simulink model "MPC_plant"  (R2024b)
settings: Solver=ode45  StartTime=0.0  StopTime=400  RelTol=1e-2  EnableMultiTasking=on
values from neighbouring files (symbols this model uses):
  alfa = [alfaa alfab alfac alfad alfae alfaf]    [dati.m]
  F0B = 0.5    [dati.m]
  F0E = u(10)    [R2_stati.m]    (also in dati.m = 99.5)
  H1 = [Hr1;He1*ones(Ne1,1);Hf1;Ha1*ones(Na1,1);Hc1]    [dati.m]
  H2 = [Hr2;He2*ones(Ne2,1);Hf2;Ha2*ones(Na2,1);Hc2]    [dati.m]
  H3 = [Hr3;He3*ones(Ne3,1);Hf3;Ha3*ones(Na3,1);Hc3]    [dati.m]
  k1 = 10    [dati.m]
  k2 = 50    [dati.m]
  N1 = Na1+Ne1+3    (= 9)    [dati.m]
  N2 = Na2+Ne2+3    (= 9)    [dati.m]
  N3 = Na3+Ne3+3    (= 9)    [dati.m]
  Na1 = 3    [dati.m]
  Na2 = 3    [dati.m]
  Na3 = 3    [dati.m]
  Ne1 = 3    [dati.m]
  Ne2 = 3    [dati.m]
  Ne3 = 3    [dati.m]
  V1 = 330+80    (= 410)    [dati.m]
  V2 = 385    [dati.m]
  V3 = 282    [dati.m]
  VR1 = 1000    [dati.m]
  VR2 = 850    [dati.m]
  x1a = zeros(N1,1)    [dati.m]
  x1b = zeros(N1,1)    [dati.m]
  x1c = zeros(N1,1)    [dati.m]
  x2a = zeros(N2,1)    [dati.m]
  x2b = zeros(N2,1)    [dati.m]
  x2c = zeros(N2,1)    [dati.m]
  x3a = zeros(N3,1)    [dati.m]
  x3b = zeros(N3,1)    [dati.m]
  x3c = zeros(N3,1)    [dati.m]
  xD3_a = 0.    (= 0)    [dati.m]
  xD3_c = 0.0036    [dati.m]
  xD3_d = 0.2817    [dati.m]
  xk0_obs = 0.5*ones(states_tot, 1)    [Initialize_forequilibrium.m]    (also in MPC_main.m)
  z0A_a = 1    [dati.m]
  z0A_b = 0    [dati.m]
  z0A_c = 0    [dati.m]
  z0A_d = 0    [dati.m]
  z0B_a = 0    [dati.m]
  z0B_b = 1    [dati.m]
  z0B_c = 0    [dati.m]
  z0B_d = 0    [dati.m]
  z0E_b = 0    [dati.m]
  z0E_d = 0    [dati.m]
  z0E_e = 1    [dati.m]
  z0E_f = 0    [dati.m]
  z1a = 0.184    [dati.m]
  z1b = 0.0544    [dati.m]
  z1c = 0.3255    [dati.m]
  z1d = 0.4361    [dati.m]
  z2b = u(4)    [R2_stati.m]    (also in R3_stati.m = u(9); dati.m = 0.4455)
  z2d = u(1)    [R2_stati.m]    (also in R3_stati.m = u(6); dati.m = 0.0514)
  z2e = u(2)    [R2_stati.m]    (also in R3_stati.m = u(7); dati.m = 0.0411)
  z2f = u(3)    [R2_stati.m]    (also in R3_stati.m = u(8); dati.m = 0.4455)
  z3b = u(4)    [R3_stati.m]    (also in dati.m = 0.4666)
  z3d = u(1)    [R3_stati.m]    (also in dati.m = 0.0523)
  z3e = u(2)    [R3_stati.m]    (also in dati.m = 0.0032)
  z3f = u(3)    [R3_stati.m]    (also in dati.m = 0.4666)
undefined symbols (not defined in the file or in its folder): colonna1, colonna2, colonna3, R1_portata, R1_stati, R2_portata, R2_stati, R3_portata, R3_stati, somma
settings Model: Creator=scattolini  LastModifiedBy=Laura
settings SolverCC: AlgebraicLoopSolver=TrustRegion
settings DataIOCC: LimitDataPoints=on  SaveFormat=Array  SignalLoggingSaveFormat=ModelDataLogs  ReturnWorkspaceOutputs=off
settings OptimizationCC: BlockReduction=off  DefaultParameterBehavior=Inlined  InlineInvariantSignals=on  BufferReuse=off  ExpressionDepthLimit=2147483647  InitFltsAndDblsToZero=on  LifeSpan=inf
settings DebuggingCC: SaveWithParameterizedLinksMsg=none  UnderspecifiedInitializationDetection=Classic  MergeDetectMultiDrivingBlocksExec=none  SignalResolutionControl=TryResolveAllWithWarning  SolverPrmCheckMsg=warning  MultiTaskDSMMsg=warning  MultiTaskCondExecSysMsg=none  FcnCallInpInsideContextMsg=warning  UnconnectedInputMsg=warning  UnconnectedOutputMsg=warning  UnconnectedLineMsg=warning  StateNameClashWarn=warning  SFUnexpectedBacktrackingDiag=warning  SFNoUnconditionalDefaultTransitionDiag=warning  SFExecutionAtInitializationDiag=none  ArithmeticOperatorsInVariantConditions=warning
settings HardwareCC: ProdBitPerPointer=32  ProdBitPerSizeT=32  ProdBitPerPtrDiffT=32  ProdLargestAtomicFloat=None  ProdIntDivRoundTo=Undefined  ProdEndianess=Unspecified  ProdWordSize=32  ProdHWDeviceType=32-bit Generic
settings ModelReferenceCC: EnableRefExpFcnMdlSchedulingChecks=on  PropagateSignalLabelsOutOfModel=off
settings RTWCC: GPUComputeCapability=3.5  DLArmComputeVersion=19.05
settings CodeAppCC: StateflowObjectComments=on
settings GRTTargetCC: TargetFcnLib=ansi_tfl_tmw.mat  TargetLangStandard=C89/C90 (ANSI)  CombineOutputUpdateFcns=off  GRTInterface=on
settings ConfigComp: CovMetricSettings=dw  CovSaveCumulativeToWorkspaceVar=on  CovSaveSingleToWorkspaceVar=on

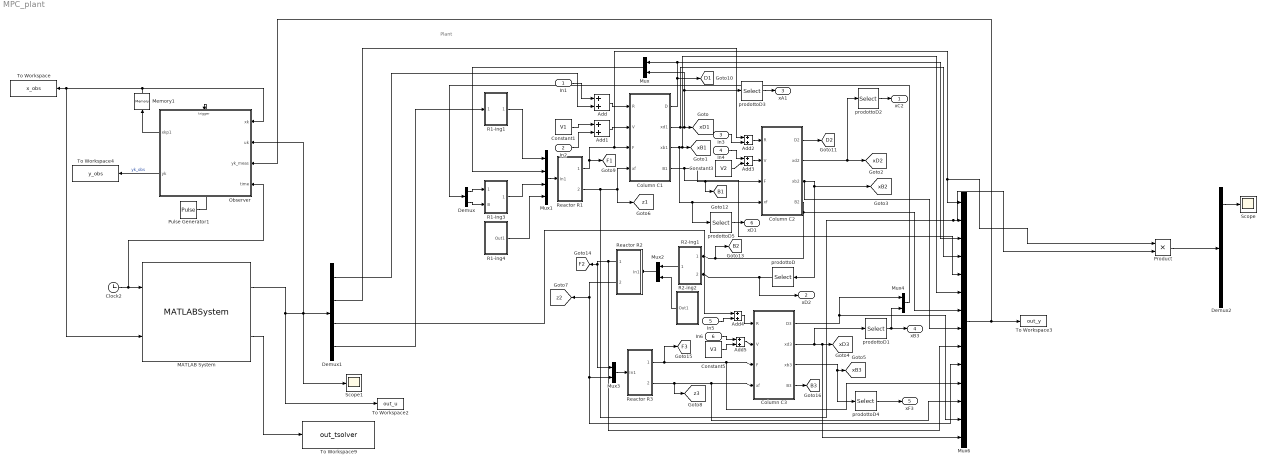
== system MPC_plant ==
  note: Plant
  In1 : Inport
  In2 : Inport  Port=2
  In3 : Inport  Port=3
  In4 : Inport  Port=4
  In5 : Inport  Port=5
  In6 : Inport  Port=6
  Add{,1..5} (6 alike) : Sum
  Clock2 : Clock
  Column C1 : Subsystem
  Column C2 : Subsystem
  Column C3 : Subsystem
  Constant1 : Constant  Value=V1
  Constant3 : Constant  Value=V2
  Constant5 : Constant  Value=V3
  Demux : Demux  Outputs=2
  Demux1 : Demux
  Demux2 : Demux
  MATLAB System : MATLABSystem  System=MPC_function  tau_s=1  N=12  T_s=1  T_b=1  SimulateUsing=Interpreted execution
      mask Type: MPC_function
      mask Display:
      | disp('MPC_function');
      | port_label('input',1,'t');
      | port_label('input',2,'xk');
      | port_label('output',1,'u_opt');
      | port_label('output',2,'t_solver');
  Memory1 : Memory  InitialCondition=xk0_obs
  Mux{,2..4} (4 alike) : Mux  Inputs=2
  Mux1 : Mux
  Mux6 : Mux  Inputs=14
  Observer : Subsystem  TreatAsAtomicUnit=on
  Product : Product
  Pulse Generator1 : DiscretePulseGenerator  PulseType=Time based  Period=1  PulseWidth=5
  R1-ing1 : Subsystem
  R1-ing3 : Subsystem
  R1-ing4 : Subsystem
  R2-ing1 : Subsystem
  R2-ing2 : Subsystem
  Reactor R1 : Subsystem
  Reactor R2 : Subsystem
  Reactor R3 : Subsystem
  Scope : Scope
  Scope1 : Scope
  To Workspace : ToWorkspace  VariableName=x_obs  SampleTime=1
  To Workspace2 : ToWorkspace  VariableName=out_u  SampleTime=1
  To Workspace3 : ToWorkspace  VariableName=out_y  SampleTime=1
  To Workspace4 : ToWorkspace  VariableName=y_obs  SampleTime=1
  To Workspace9 : ToWorkspace  VariableName=out_tsolver  SampleTime=1
  prodottoD : Selector  InputPortWidth=4  IndexOptions=Index vector (dialog)  Indices=4  OutputSizes=1
  prodottoD1 : Selector  InputPortWidth=4  IndexOptions=Index vector (dialog)  Indices=1  OutputSizes=1
  prodottoD2 : Selector  InputPortWidth=4  IndexOptions=Index vector (dialog)  Indices=3  OutputSizes=1
  prodottoD3 : Selector  InputPortWidth=4  IndexOptions=Index vector (dialog)  Indices=1  OutputSizes=1
  prodottoD4 : Selector  InputPortWidth=4  IndexOptions=Index vector (dialog)  Indices=4  OutputSizes=1
  prodottoD5 : Selector  InputPortWidth=4  IndexOptions=Index vector (dialog)  Indices=4  OutputSizes=1
  xC2 : Outport
  xD2 : Outport  Port=2
  xA1 : Outport  Port=3
  xB3 : Outport  Port=4
  xF3 : Outport  Port=5
  xD1 : Outport  Port=6
  tag scope: B1=global, B2=global, B3=global, D1=global, D2=global, F1=global, F2=global, F3=global, xB1=global, xB2=global, xB3=global, xD1=global, xD2=global, xD3=global, z1=global, z2=global, z3=global
  wires:
  R1-ing1/1(Out1) -> Mux1/1
  R1-ing3/1(Out1) -> Mux1/3
  R1-ing4/1(Out1) -> Mux1/4
  Mux1/1 -> Reactor R1/1(In1)
  Column C1/3(xb1) -> Mux6/6, [xB1], Column C2/4(xf), prodottoD5/1
  Column C1/2(xd1) -> Mux6/4, [xD1], Mux/2, prodottoD3/1
  Column C1/1(D) -> Mux6/3, Mux/1, [D1]
  Mux/1 -> Mux1/2
  Column C1/4(B1) -> Mux6/5, Column C2/3(F), [B1]
  prodottoD/1 -> R2-ing1/2(prodottoD), xD2/1
  Mux2/1 -> Reactor R2/1(In1)
  R2-ing1/1(Out1) -> Mux2/1
  R2-ing2/1(Out1) -> Mux2/2
  Reactor R2/2(stati) -> Mux6/10, Mux3/2, [z2]
  Reactor R2/1(portata) -> Mux6/9, Mux3/1, [F2]
  Mux3/1 -> Reactor R3/1(In1)
  Reactor R3/1(portata) -> Mux6/11, Column C3/3(F), [F3]
  Reactor R3/2(stati B-D-E-F) -> Mux6/12, Column C3/4(xf), [z3]
  Column C3/3(xb3) -> [xB3], prodottoD4/1
  Column C3/2(xd3) -> Mux6/14, [xD3], prodottoD1/1
  Column C2/2(xd2) -> [xD2], prodottoD2/1
  Column C2/1(D2) -> [D2]
  prodottoD1/1 -> Mux4/2, xB3/1
  Column C3/1(D3) -> Mux4/1, Mux6/13
  Mux4/1 -> Demux/1
  Demux/1 -> R1-ing3/1(portata)
  Demux/2 -> R1-ing3/2(B)
  Demux1/1 -> Add/2
  In1/1 -> Add/1
  Add/1 -> Column C1/1(R)
  prodottoD2/1 -> xC2/1
  Add1/1 -> Column C1/2(V)
  Constant1/1 -> Add1/1
  In2/1 -> Add1/2
  Add2/1 -> Column C2/1(R)
  Add3/1 -> Column C2/2(V)
  Constant3/1 -> Add3/2
  In3/1 -> Add2/2
  In4/1 -> Add3/1
  prodottoD3/1 -> xA1/1
  Add5/1 -> Column C3/2(V)
  Constant5/1 -> Add5/2
  In6/1 -> Add5/1
  In5/1 -> Add4/2
  prodottoD4/1 -> xF3/1
  Column C3/4(B3) -> [B3]
  Add4/1 -> Column C3/1(R)
  prodottoD5/1 -> xD1/1
  Mux6/1 -> Observer/3(yk_meas), To Workspace3/1
  Pulse Generator1/1 -> Observer/Trigger
  Observer/1(xkp1) -> Memory1/1
  Memory1/1 -> Observer/1(xk), To Workspace/1, MATLAB System/2
  Observer/2(yk) -> To Workspace4/1  "yk_obs"
  Column C2/3(xb2) -> Mux6/8, prodottoD/1, [xB2]
  Column C2/4(B2) -> Mux6/7, R2-ing1/1(portataD), [B2]
  Clock2/1 -> Observer/4(time), MATLAB System/1
  Demux1/2 -> Add2/1
  Demux1/3 -> Add4/1
  Demux1/4 -> R1-ing1/1(F0A)
  Reactor R1/1(portata) -> Mux6/1, Product/1, Column C1/3(F), [F1]
  Reactor R1/2(stati) -> Product/2, Mux6/2, Column C1/4(xf), [z1]
  Product/1 -> Demux2/1
  Demux2/1 -> Scope/1
  MATLAB System/1 -> To Workspace2/1, Demux1/1, Observer/2(uk), Scope1/1
  MATLAB System/2 -> To Workspace9/1

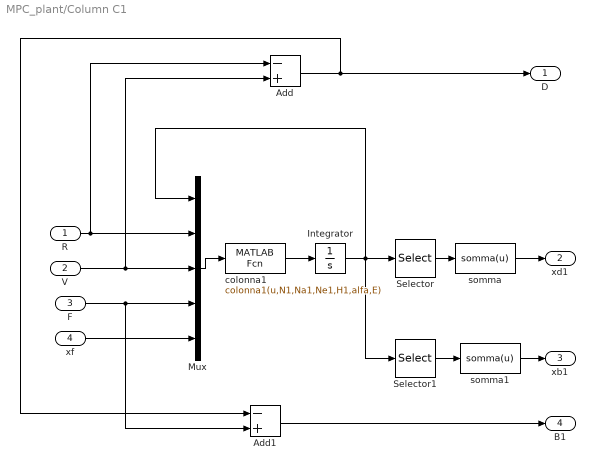
== system MPC_plant/Column C1 ==
  R : Inport
  V : Inport  Port=2
  F : Inport  Port=3
  xf : Inport  Port=4
  Add : Sum  Inputs=-+
  Add1 : Sum  Inputs=-+
  Integrator : Integrator  InitialCondition=[x1a;x1b;x1c]
  Mux : Mux  Inputs=5
  Selector : Selector  InputPortWidth=N1*3  IndexOptions=Index vector (dialog)  Indices=[N1 2*N1 3*N1]  OutputSizes=1
  Selector1 : Selector  InputPortWidth=N1*3  IndexOptions=Index vector (dialog)  Indices=[1 N1+1 2*N1+1]  OutputSizes=1
  colonna1 : MATLABFcn  MATLABFcn=colonna1(u,N1,Na1,Ne1,H1,alfa,E)  OutputDimensions=N1*3
  somma : MATLABFcn  MATLABFcn=somma(u)  OutputDimensions=4
  somma1 : MATLABFcn  MATLABFcn=somma(u)  OutputDimensions=4
  D : Outport
  xd1 : Outport  Port=2
  xb1 : Outport  Port=3
  B1 : Outport  Port=4
  wires:
  Mux/1 -> colonna1/1
  colonna1/1 -> Integrator/1
  Integrator/1 -> Selector/1, Mux/1, Selector1/1
  R/1 -> Mux/2, Add/1
  V/1 -> Mux/3, Add/2
  F/1 -> Mux/4, Add1/2
  xf/1 -> Mux/5
  Selector/1 -> somma/1
  somma/1 -> xd1/1
  Selector1/1 -> somma1/1
  somma1/1 -> xb1/1
  Add/1 -> D/1, Add1/1
  Add1/1 -> B1/1

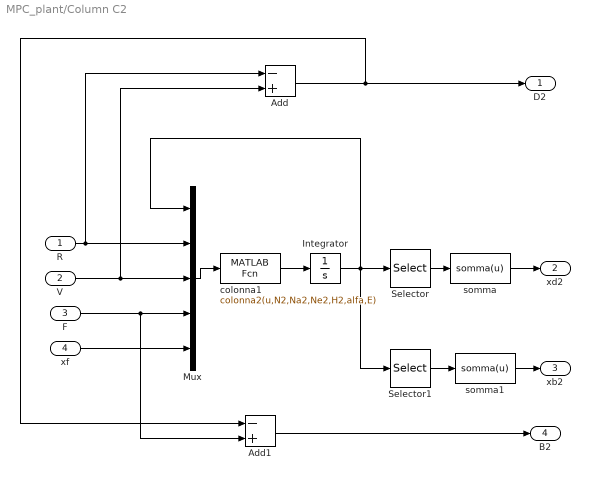
== system MPC_plant/Column C2 ==
  R : Inport
  V : Inport  Port=2
  F : Inport  Port=3
  xf : Inport  Port=4
  Add : Sum  Inputs=-+
  Add1 : Sum  Inputs=-+
  Integrator : Integrator  InitialCondition=[x2a;x2b;x2c]
  Mux : Mux  Inputs=5
  Selector : Selector  InputPortWidth=N2*3  IndexOptions=Index vector (dialog)  Indices=[N2 2*N2 3*N2]  OutputSizes=1
  Selector1 : Selector  InputPortWidth=N2*3  IndexOptions=Index vector (dialog)  Indices=[1 N2+1 2*N2+1]  OutputSizes=1
  colonna1 : MATLABFcn  MATLABFcn=colonna2(u,N2,Na2,Ne2,H2,alfa,E)  OutputDimensions=N2*3
  somma : MATLABFcn  MATLABFcn=somma(u)  OutputDimensions=4
  somma1 : MATLABFcn  MATLABFcn=somma(u)  OutputDimensions=4
  D2 : Outport
  xd2 : Outport  Port=2
  xb2 : Outport  Port=3
  B2 : Outport  Port=4
  wires:
  Mux/1 -> colonna1/1
  colonna1/1 -> Integrator/1
  Integrator/1 -> Selector/1, Mux/1, Selector1/1
  R/1 -> Mux/2, Add/1
  V/1 -> Mux/3, Add/2
  F/1 -> Mux/4, Add1/2
  xf/1 -> Mux/5
  Selector/1 -> somma/1
  somma/1 -> xd2/1
  Selector1/1 -> somma1/1
  somma1/1 -> xb2/1
  Add/1 -> D2/1, Add1/1
  Add1/1 -> B2/1

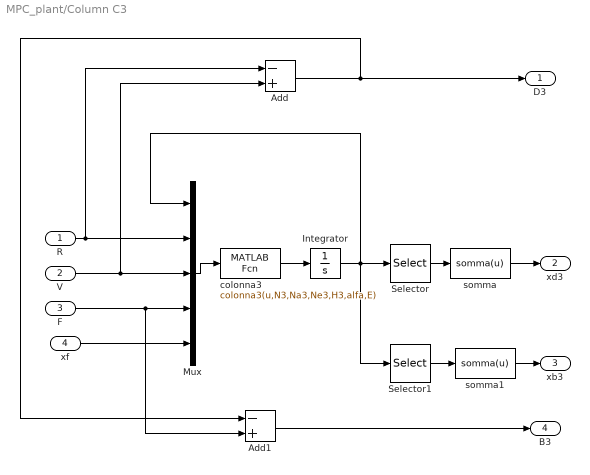
== system MPC_plant/Column C3 ==
  R : Inport
  V : Inport  Port=2
  F : Inport  Port=3
  xf : Inport  Port=4
  Add : Sum  Inputs=-+
  Add1 : Sum  Inputs=-+
  Integrator : Integrator  InitialCondition=[x3a;x3b;x3c]
  Mux : Mux  Inputs=5
  Selector : Selector  InputPortWidth=N3*3  IndexOptions=Index vector (dialog)  Indices=[N3 2*N3 3*N3]  OutputSizes=1
  Selector1 : Selector  InputPortWidth=N3*3  IndexOptions=Index vector (dialog)  Indices=[1 N3+1 2*N3+1]  OutputSizes=1
  colonna3 : MATLABFcn  MATLABFcn=colonna3(u,N3,Na3,Ne3,H3,alfa,E)  OutputDimensions=N3*3
  somma : MATLABFcn  MATLABFcn=somma(u)  OutputDimensions=4
  somma1 : MATLABFcn  MATLABFcn=somma(u)  OutputDimensions=4
  D3 : Outport
  xd3 : Outport  Port=2
  xb3 : Outport  Port=3
  B3 : Outport  Port=4
  wires:
  Mux/1 -> colonna3/1
  colonna3/1 -> Integrator/1
  Integrator/1 -> Selector/1, Mux/1, Selector1/1
  R/1 -> Mux/2, Add/1
  V/1 -> Mux/3, Add/2
  F/1 -> Mux/4, Add1/2
  xf/1 -> Mux/5
  Selector/1 -> somma/1
  somma/1 -> xd3/1
  Selector1/1 -> somma1/1
  somma1/1 -> xb3/1
  Add/1 -> D3/1, Add1/1
  Add1/1 -> B3/1

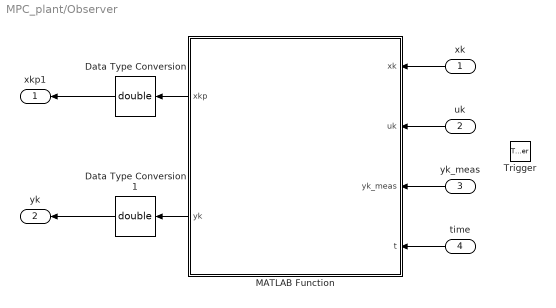
== system MPC_plant/Observer ==
  xk : Inport
  uk : Inport  Port=2
  yk_meas : Inport  Port=3
  time : Inport  Port=4
  Trigger : TriggerPort  VariantControl=(inherit)
  Data Type Conversion : DataTypeConversion  OutDataTypeStr=double  RndMeth=Nearest  SaturateOnIntegerOverflow=off
  Data Type Conversion1 : DataTypeConversion  OutDataTypeStr=double  RndMeth=Nearest  SaturateOnIntegerOverflow=off
  MATLAB Function : MATLAB Function  TreatAsAtomicUnit=on
  xkp1 : Outport
  yk : Outport  Port=2
  wires:
  xk/1 -> MATLAB Function/1(xk)
  uk/1 -> MATLAB Function/2(uk)
  MATLAB Function/2(yk) -> Data Type Conversion1/1
  MATLAB Function/1(xkp) -> Data Type Conversion/1
  Data Type Conversion/1 -> xkp1/1
  Data Type Conversion1/1 -> yk/1
  yk_meas/1 -> MATLAB Function/3(yk_meas)
  time/1 -> MATLAB Function/4(t)

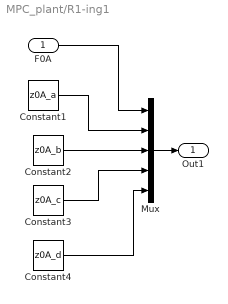
== system MPC_plant/R1-ing1 ==
  F0A : Inport
  Constant1 : Constant  Value=z0A_a
  Constant2 : Constant  Value=z0A_b
  Constant3 : Constant  Value=z0A_c
  Constant4 : Constant  Value=z0A_d
  Mux : Mux  Inputs=5
  Out1 : Outport
  wires:
  Constant1/1 -> Mux/2
  Constant2/1 -> Mux/3
  Constant3/1 -> Mux/4
  Constant4/1 -> Mux/5
  Mux/1 -> Out1/1
  F0A/1 -> Mux/1

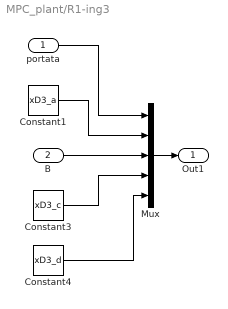
== system MPC_plant/R1-ing3 ==
  portata : Inport
  B : Inport  Port=2
  Constant1 : Constant  Value=xD3_a
  Constant3 : Constant  Value=xD3_c
  Constant4 : Constant  Value=xD3_d
  Mux : Mux  Inputs=5
  Out1 : Outport
  wires:
  portata/1 -> Mux/1
  Constant1/1 -> Mux/2
  B/1 -> Mux/3
  Constant3/1 -> Mux/4
  Constant4/1 -> Mux/5
  Mux/1 -> Out1/1

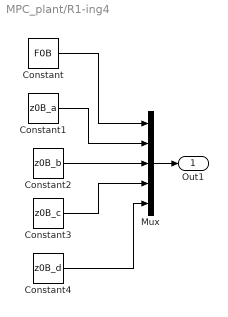
== system MPC_plant/R1-ing4 ==
  Constant : Constant  Value=F0B
  Constant1 : Constant  Value=z0B_a
  Constant2 : Constant  Value=z0B_b
  Constant3 : Constant  Value=z0B_c
  Constant4 : Constant  Value=z0B_d
  Mux : Mux  Inputs=5
  Out1 : Outport
  wires:
  Constant/1 -> Mux/1
  Constant1/1 -> Mux/2
  Constant2/1 -> Mux/3
  Constant3/1 -> Mux/4
  Constant4/1 -> Mux/5
  Mux/1 -> Out1/1

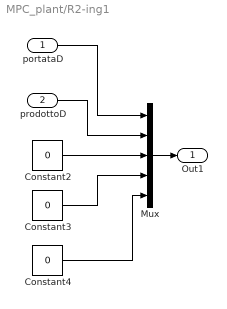
== system MPC_plant/R2-ing1 ==
  portataD : Inport
  prodottoD : Inport  Port=2
  Constant2 : Constant  Value=0
  Constant3 : Constant  Value=0
  Constant4 : Constant  Value=0
  Mux : Mux  Inputs=5
  Out1 : Outport
  wires:
  portataD/1 -> Mux/1
  prodottoD/1 -> Mux/2
  Constant2/1 -> Mux/3
  Constant3/1 -> Mux/4
  Constant4/1 -> Mux/5
  Mux/1 -> Out1/1

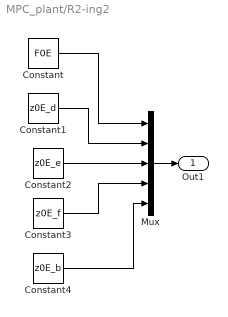
== system MPC_plant/R2-ing2 ==
  Constant : Constant  Value=F0E
  Constant1 : Constant  Value=z0E_d
  Constant2 : Constant  Value=z0E_e
  Constant3 : Constant  Value=z0E_f
  Constant4 : Constant  Value=z0E_b
  Mux : Mux  Inputs=5
  Out1 : Outport
  wires:
  Constant/1 -> Mux/1
  Constant1/1 -> Mux/2
  Constant2/1 -> Mux/3
  Constant3/1 -> Mux/4
  Constant4/1 -> Mux/5
  Mux/1 -> Out1/1

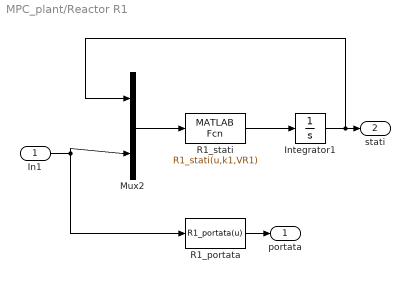
== system MPC_plant/Reactor R1 ==
  In1 : Inport
  Integrator1 : Integrator  InitialCondition=[z1a z1b z1c z1d]
  Mux2 : Mux  Inputs=2
  R1_portata : MATLABFcn  MATLABFcn=R1_portata(u)
  R1_stati : MATLABFcn  MATLABFcn=R1_stati(u,k1,VR1)  OutputDimensions=4
  portata : Outport
  stati : Outport  Port=2
  wires:
  In1/1 -> Mux2/2, R1_portata/1
  R1_stati/1 -> Integrator1/1
  Mux2/1 -> R1_stati/1
  Integrator1/1 -> Mux2/1, stati/1
  R1_portata/1 -> portata/1

== system MPC_plant/Reactor R2 ==
  In1 : Inport
  Integrator1 : Integrator  InitialCondition=[z2d z2e z2f z2b]
  Mux2 : Mux  Inputs=2
  R2_portata : MATLABFcn  MATLABFcn=R2_portata(u)
  R2_stati : MATLABFcn  MATLABFcn=R2_stati(u,k2,VR2)  OutputDimensions=4
  portata : Outport
  stati : Outport  Port=2
  wires:
  In1/1 -> Mux2/2, R2_portata/1
  R2_stati/1 -> Integrator1/1
  Mux2/1 -> R2_stati/1
  Integrator1/1 -> Mux2/1, stati/1
  R2_portata/1 -> portata/1

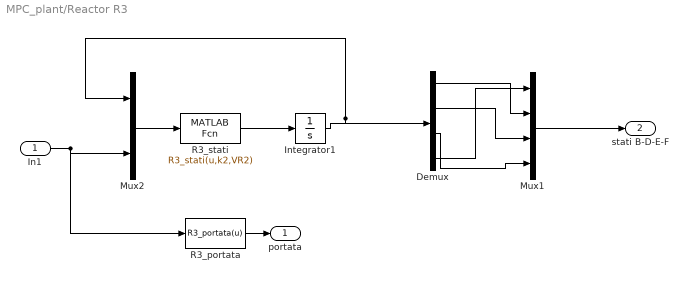
== system MPC_plant/Reactor R3 ==
  In1 : Inport
  Demux : Demux
  Integrator1 : Integrator  InitialCondition=[z3d z3e z3f z3b]
  Mux1 : Mux
  Mux2 : Mux  Inputs=2
  R3_portata : MATLABFcn  MATLABFcn=R3_portata(u)
  R3_stati : MATLABFcn  MATLABFcn=R3_stati(u,k2,VR2)  OutputDimensions=4
  portata : Outport
  stati B-D-E-F : Outport  Port=2
  wires:
  In1/1 -> Mux2/2, R3_portata/1
  R3_stati/1 -> Integrator1/1
  Mux2/1 -> R3_stati/1
  Integrator1/1 -> Mux2/1, Demux/1
  R3_portata/1 -> portata/1
  Demux/4 -> Mux1/1
  Demux/1 -> Mux1/2
  Demux/2 -> Mux1/3
  Demux/3 -> Mux1/4
  Mux1/1 -> stati B-D-E-F/1

== matlab function MPC_plant/Observer/MATLAB Function ==
  data: xkp output; xk input; uk input; yk_meas input; t input; yk output
function [xkp, yk] = RNN(xk, uk, yk_meas, t)

    if t <= 1
        xk = 0.5*ones(18, 1);
    end

    n_states = [3,3,3,3,3,3];
    layers_file = load("layers_file.mat");
    layers_file = layers_file.layers_file;
    input_scaler_bias = load("input_scaler_bias.mat");
    input_scaler_scale_common = load("input_scaler_scale_common.mat");
    output_scaler_bias = load("output_scaler_bias.mat");
    output_scaler_scale_common = load("output_scaler_scale_common.mat");
    
    % Best observer weight
    Lz1_sol = load("Lz1_sol.mat");
    Lf1_sol = load("Lf1_sol.mat");
    Lz1 = Lz1_sol.Lz1;
    Lf1 = Lf1_sol.Lf1;
    Lz2_sol = load("Lz2_sol.mat");
    Lf2_sol = load("Lf2_sol.mat");
    Lz2 = Lz2_sol.Lz2;
    Lf2 = Lf2_sol.Lf2;
    Lz3_sol = load("Lz3_sol.mat");
    Lf3_sol = load("Lf3_sol.mat");
    Lz3 = Lz3_sol.Lz3;
    Lf3 = Lf3_sol.Lf3;
    Lz4_sol = load("Lz4_sol.mat");
    Lf4_sol = load("Lf4_sol.mat");
    Lz4 = Lz4_sol.Lz4;
    Lf4 = Lf4_sol.Lf4;
    Lz5_sol = load("Lz5_sol.mat");
    Lf5_sol = load("Lf5_sol.mat");
    Lz5 = Lz5_sol.Lz5;
    Lf5 = Lf5_sol.Lf5;
    Lz6_sol = load("Lz6_sol.mat");
    Lf6_sol = load("Lf6_sol.mat");
    Lz6 = Lz6_sol.Lz6;
    Lf6 = Lf6_sol.Lf6;

    % Scale input and output
    uk = (uk  - (input_scaler_bias.input_scaler_bias).') ./ (input_scaler_scale_common.input_scaler_scale_common).';
    yk_meas = [yk_meas(1)*yk_meas(2); yk_meas(1)*yk_meas(3); yk_meas(1)*yk_meas(4); yk_meas(1)*yk_meas(5); yk_meas(6)*yk_meas(7); yk_meas(6)*yk_meas(8); yk_meas(6)*yk_meas(9); yk_meas(6)*yk_meas(10); yk_meas(11)*yk_meas(12); yk_meas(11)*yk_meas(13); yk_meas(11)*yk_meas(14); yk_meas(11)*yk_meas(15); yk_meas(16)*yk_meas(17); yk_meas(11)*yk_meas(18); yk_meas(11)*yk_meas(19); yk_meas(11)*yk_meas(20); yk_meas(21)*yk_meas(22); yk_meas(21)*yk_meas(23); yk_meas(21)*yk_meas(24); yk_meas(21)*yk_meas(25); yk_meas(26)*yk_meas(27); yk_meas(26)*yk_meas(28); yk_meas(26)*yk_meas(29); yk_meas(26)*yk_meas(30); yk_meas(31)*yk_meas(32); yk_meas(31)*yk_meas(33); yk_meas(31)*yk_meas(34); yk_meas(31)*yk_meas(35)];
    yk_meas = (yk_meas  - (output_scaler_bias.output_scaler_bias).') ./ (output_scaler_scale_common.output_scaler_scale_common).';

    % GRU 1
    yk1_meas = yk_meas(1:4,:);
    yk2_to1_meas = yk_meas(5:8,:);
    yk6_meas = yk_meas(25:28,:);
    uk1 = [uk(1,:); uk(3:4,:); yk2_to1_meas; yk6_meas];
    xk1 = xk(1:n_states(1),:);    
    yk1 = layers_file.layers{1,2}.weights.weight * xk1 + (layers_file.layers{1,2}.weights.bias).';
    zk1 = sigmoidfunction((layers_file.layers{1,1}.weights.Wzf(:,1:n_states(1))).' * uk1 + (layers_file.layers{1,1}.weights.Uzf(:,1:n_states(1))).' * xk1 + (layers_file.layers{1,1}.weights.bzf(:,1:n_states(1))).' + Lz1*(yk1_meas-yk1) );
    fk1 = sigmoidfunction((layers_file.layers{1,1}.weights.Wzf(:,n_states(1)+1:end)).' * uk1 + (layers_file.layers{1,1}.weights.Uzf(:,n_states(1)+1:end)).' * xk1 + (layers_file.layers{1,1}.weights.bzf(:,n_states(1)+1:end)).' + Lf1*(yk1_meas-yk1) );
    phi1 = tanh((layers_file.layers{1,1}.weights.Wr).' * uk1 + (layers_file.layers{1,1}.weights.Ur).' * (fk1.* xk1) + (layers_file.layers{1,1}.weights.br).');
    xkp1 = zk1 .* xk1 + (1-zk1) .* phi1;
    
    % GRU 2    
    yk2_meas = yk_meas(5:12,:);
    yk2_to3_meas = yk_meas(9:12,:);
    uk2 = [uk(1,:); uk(3:4,:); yk1_meas];
    xk2 = xk(n_states(1)+1:n_states(1)+n_states(2),:);
    yk2 = layers_file.layers{1,4}.weights.weight * xk2 + (layers_file.layers{1,4}.weights.bias).';
    zk2 = sigmoidfunction((layers_file.layers{1,3}.weights.Wzf(:,1:n_states(2))).' * uk2 + (layers_file.layers{1,3}.weights.Uzf(:,1:n_states(2))).' * xk2 + (layers_file.layers{1,3}.weights.bzf(:,1:n_states(2))).' + Lz2*(yk2_meas-yk2) );
    fk2 = sigmoidfunction((layers_file.layers{1,3}.weights.Wzf(:,n_states(2)+1:end)).' * uk2 + (layers_file.layers{1,3}.weights.Uzf(:,n_states(2)+1:end)).' * xk2 + (layers_file.layers{1,3}.weights.bzf(:,n_states(2)+1:end)).' + Lf2*(yk2_meas-yk2) );
    phi2 = tanh((layers_file.layers{1,3}.weights.Wr).' * uk2 + (layers_file.layers{1,3}.weights.Ur).' * (fk2.* xk2) + (layers_file.layers{1,3}.weights.br).');
    xkp2 = zk2 .* xk2 + (1-zk2) .* phi2;
    
    % GRU 3
    yk3_meas = yk_meas(13:16,:);
    uk3 = [uk(2:4,:); yk2_to3_meas];
    xk3 = xk(n_states(1)+n_states(2)+1:n_states(1)+n_states(2)+n_states(3),:);
    yk3 = layers_file.layers{1,6}.weights.weight * xk3 + (layers_file.layers{1,6}.weights.bias).';
    zk3 = sigmoidfunction((layers_file.layers{1,5}.weights.Wzf(:,1:n_states(3))).' * uk3 + (layers_file.layers{1,5}.weights.Uzf(:,1:n_states(3))).' * xk3 + (layers_file.layers{1,5}.weights.bzf(:,1:n_states(3))).' + Lz3*(yk3_meas-yk3) );
    fk3 = sigmoidfunction((layers_file.layers{1,5}.weights.Wzf(:,n_states(3)+1:end)).' * uk3 + (layers_file.layers{1,5}.weights.Uzf(:,n_states(3)+1:end)).' * xk3 + (layers_file.layers{1,5}.weights.bzf(:,n_states(3)+1:end)).' + Lf3*(yk3_meas-yk3) );
    phi3 = tanh((layers_file.layers{1,5}.weights.Wr).' * uk3 + (layers_file.layers{1,5}.weights.Ur).' * (fk3.* xk3) + (layers_file.layers{1,5}.weights.br).');
    xkp3 = zk3 .* xk3 + (1-zk3) .* phi3;

    % GRU 4
    yk4_meas = yk_meas(17:20,:);
    uk4 = [uk(2:4,:); yk3_meas];
    xk4 = xk(n_states(1)+n_states(2)+n_states(3)+1:n_states(1)+n_states(2)+n_states(3)+n_states(4),:);
    yk4 = layers_file.layers{1,8}.weights.weight * xk4 + (layers_file.layers{1,8}.weights.bias).';
    zk4 = sigmoidfunction((layers_file.layers{1,7}.weights.Wzf(:,1:n_states(4))).' * uk4 + (layers_file.layers{1,7}.weights.Uzf(:,1:n_states(4))).' * xk4 + (layers_file.layers{1,7}.weights.bzf(:,1:n_states(4))).' + Lz4*(yk4_meas-yk4) );
    fk4 = sigmoidfunction((layers_file.layers{1,7}.weights.Wzf(:,n_states(4)+1:end)).' * uk4 + (layers_file.layers{1,7}.weights.Uzf(:,n_states(4)+1:end)).' * xk4 + (layers_file.layers{1,7}.weights.bzf(:,n_states(4)+1:end)).' + Lf4*(yk4_meas-yk4) );
    phi4 = tanh((layers_file.layers{1,7}.weights.Wr).' * uk4 + (layers_file.layers{1,7}.weights.Ur).' * (fk4.* xk4) + (layers_file.layers{1,7}.weights.br).');
    xkp4 = zk4 .* xk4 + (1-zk4) .* phi4;

    % GRU 5
    yk5_meas = yk_meas(21:24,:);
    uk5 = [uk(2:4,:); yk4_meas];
    xk5 = xk(n_states(1)+n_states(2)+n_states(3)+n_states(4)+1:n_states(1)+n_states(2)+n_states(3)+n_states(4)+n_states(5),:);
    yk5 = layers_file.layers{1,10}.weights.weight * xk5 + (layers_file.layers{1,10}.weights.bias).';
    zk5 = sigmoidfunction((layers_file.layers{1,9}.weights.Wzf(:,1:n_states(5))).' * uk5 + (layers_file.layers{1,9}.weights.Uzf(:,1:n_states(5))).' * xk5 + (layers_file.layers{1,9}.weights.bzf(:,1:n_states(5))).' + Lz5*(yk5_meas-yk5) );
    fk5 = sigmoidfunction((layers_file.layers{1,9}.weights.Wzf(:,n_states(5)+1:end)).' * uk5 + (layers_file.layers{1,9}.weights.Uzf(:,n_states(5)+1:end)).' * xk5 + (layers_file.layers{1,9}.weights.bzf(:,n_states(5)+1:end)).' + Lf5*(yk5_meas-yk5) );
    phi5 = tanh((layers_file.layers{1,9}.weights.Wr).' * uk5 + (layers_file.layers{1,9}.weights.Ur).' * (fk5.* xk5) + (layers_file.layers{1,9}.weights.br).');
    xkp5 = zk5 .* xk5 + (1-zk5) .* phi5;

    % GRU 6
    uk6 = [uk(2:4,:); yk5_meas];
    xk6 = xk(n_states(1)+n_states(2)+n_states(3)+n_states(4)+n_states(5)+1:n_states(1)+n_states(2)+n_states(3)+n_states(4)+n_states(5)+n_states(6),:);
    yk6 = layers_file.layers{1,12}.weights.weight * xk6 + (layers_file.layers{1,12}.weights.bias).';
    zk6 = sigmoidfunction((layers_file.layers{1,11}.weights.Wzf(:,1:n_states(6))).' * uk6 + (layers_file.layers{1,11}.weights.Uzf(:,1:n_states(6))).' * xk6 + (layers_file.layers{1,11}.weights.bzf(:,1:n_states(6))).' + Lz6*(yk6_meas-yk6) );
    fk6 = sigmoidfunction((layers_file.layers{1,11}.weights.Wzf(:,n_states(6)+1:end)).' * uk6 + (layers_file.layers{1,11}.weights.Uzf(:,n_states(6)+1:end)).' * xk6 + (layers_file.layers{1,11}.weights.bzf(:,n_states(6)+1:end)).' + Lf6*(yk6_meas-yk6) );
    phi6 = tanh((layers_file.layers{1,11}.weights.Wr).' * uk6 + (layers_file.layers{1,11}.weights.Ur).' * (fk6.* xk6) + (layers_file.layers{1,11}.weights.br).');
    xkp6 = zk6 .* xk6 + (1-zk6) .* phi6;
    
    % Overall
    xkp = [xkp1; xkp2; xkp3; xkp4; xkp5; xkp6];
    yk = [yk1; yk2; yk3; yk4; yk5; yk6];
    yk = yk .* (output_scaler_scale_common.output_scaler_scale_common).' + (output_scaler_bias.output_scaler_bias).';
end
